simulink model "sampleModel267"  (R2021b)
settings: Solver=VariableStepAuto  StartTime=0.0  StopTime=10.0  RelTol=1e-3
undefined symbols (not defined in the file or in its folder): DiscIntNeverNeededParam, Newton, Raphson
libraries: simulink x5, slpidlib x1
settings Model: Creator=user  LastModifiedBy=user

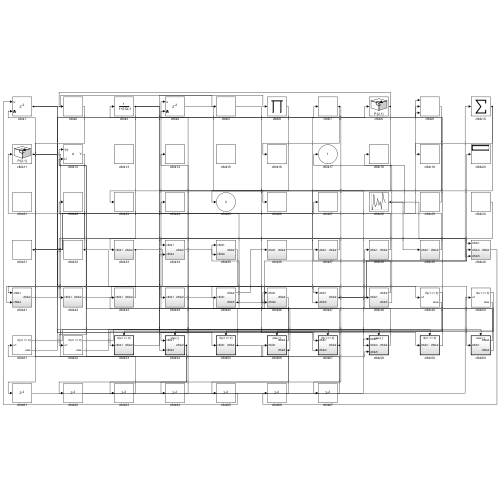
[thumbnail: Simulink's stored preview of the top-level diagram]
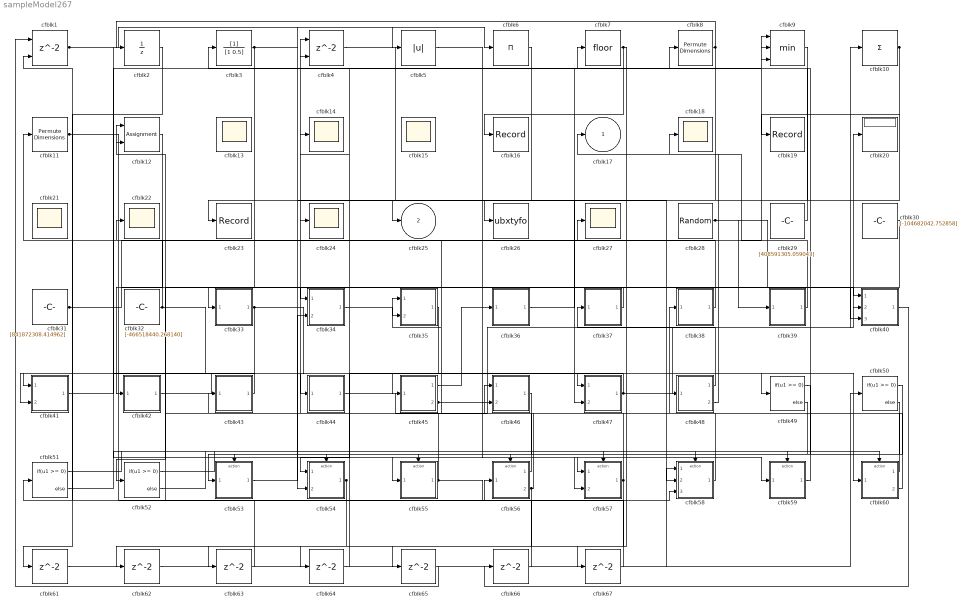
== system sampleModel267 ==
  cfblk1 : Delay  ShowEnablePort=on  SampleTime=1
      settings: InputPortMap=u0,e6
  cfblk10 : Sum  Inputs=+
  cfblk11 : PermuteDimensions
  cfblk12 : Assignment  DiagnosticForDimensions=Warning  IndexOptions=Index vector (dialog)  Indices=1  OutputSizes=1
  cfblk{13..15,18,21..22,24,27} (8 alike) : Scope
      cfblk13 settings: Floating=on
      cfblk15 settings: Floating=on
      cfblk21 settings: Floating=on
  cfblk16 : Record  FileSettingsInternal="{\"entries\":[{\"content\":{\"excelSettings\":{\"content\":{},\"type\":\"Streamout.ExcelSettings\"}},\"type\":\"Streamout.FileSettingStorage\",\"uuid\":\"38ef153d-d6ae-45e7-82f1-1ca2e326c5eb\"}],\"packageUris\":[\"http://schema.mathworks.com/mf0/streamout_blocks/R2020a\"],\"version\":\"1.0\"}"  SignalsInternal="{\"entries\":[{\"content\":{\"signals\":[{\"content\":{\"blockPath\":[\"sampleModel267/cfblk16\"],\"channel\":[],\"dimensions\":[1],\"domain\":\"sampleModel267/cfblk16\",\"lineColor\":\"#d95319\",\"plots\":[1],\"port\":1,\"sid\":[\"\"],\"signalID\":11134,\"signalName\":\"cfblk7\"},\"type\":\"RecordBlkView.Signal\",\"uuid\":\"f5056942-7931-4c3f-87a4-53e35f3bb4b1\"}]},\"type\":\"RecordBlkView.InputSignals\",\"uuid\":\"7db35bab-36c3-4b73-9a92-ac3f675e200d\"}],\"packageUris\":[\"http://schema.mathworks.com/mf0/streamout_blocks/R2020a\"],\"version\":\"1.0\"}"  VisualizationBindings="{\"sparklinesplugin\":{\"info\":[{\"bindingParametersList\":[],\"subplotID\":1}]}}"
  cfblk19 : Record  FileSettingsInternal="{\"entries\":[{\"content\":{\"excelSettings\":{\"content\":{},\"type\":\"Streamout.ExcelSettings\"}},\"type\":\"Streamout.FileSettingStorage\",\"uuid\":\"e67b9910-70a3-4f08-b618-b13b58853db8\"}],\"packageUris\":[\"http://schema.mathworks.com/mf0/streamout_blocks/R2020a\"],\"version\":\"1.0\"}"  SignalsInternal="{\"entries\":[{\"content\":{\"signals\":[{\"content\":{\"blockPath\":[\"sampleModel267/cfblk19\"],\"channel\":[],\"dimensions\":[1],\"domain\":\"sampleModel267/cfblk19\",\"lineColor\":\"#edb120\",\"plots\":[1],\"port\":1,\"sid\":[\"\"],\"signalID\":11138,\"signalName\":\"cfblk10\"},\"type\":\"RecordBlkView.Signal\",\"uuid\":\"ad1882d4-40aa-4b95-a06e-3b82c8a17900\"}]},\"type\":\"RecordBlkView.InputSignals\",\"uuid\":\"f4741eb0-9131-4b04-bfe2-4320a4acd3c2\"}],\"packageUris\":[\"http://schema.mathworks.com/mf0/streamout_blocks/R2020a\"],\"version\":\"1.0\"}"  VisualizationBindings="{\"sparklinesplugin\":{\"info\":[{\"bindingParametersList\":[],\"subplotID\":1}]}}"
  cfblk2 : UnitDelay  HasFrameUpgradeWarning=on
  cfblk20 : Display
  cfblk23 : Record  FileSettingsInternal="{\"entries\":[{\"content\":{\"excelSettings\":{\"content\":{},\"type\":\"Streamout.ExcelSettings\"}},\"type\":\"Streamout.FileSettingStorage\",\"uuid\":\"5cac87e1-3c50-4b70-acf6-de645cdb8377\"}],\"packageUris\":[\"http://schema.mathworks.com/mf0/streamout_blocks/R2020a\"],\"version\":\"1.0\"}"  SignalsInternal="{\"entries\":[{\"content\":{\"signals\":[{\"content\":{\"blockPath\":[\"sampleModel267/cfblk23\"],\"channel\":[],\"dimensions\":[1],\"domain\":\"sampleModel267/cfblk23\",\"lineColor\":\"#7e2f8e\",\"plots\":[1],\"port\":1,\"sid\":[\"\"],\"signalID\":11142,\"signalName\":\"cfblk10\"},\"type\":\"RecordBlkView.Signal\",\"uuid\":\"43345d3a-b4ac-4ed1-88fb-152ae4781999\"}]},\"type\":\"RecordBlkView.InputSignals\",\"uuid\":\"60e12632-78ef-4a34-abc7-bf1c9a5d24da\"}],\"packageUris\":[\"http://schema.mathworks.com/mf0/streamout_blocks/R2020a\"],\"version\":\"1.0\"}"  VisualizationBindings="{\"sparklinesplugin\":{\"info\":[{\"bindingParametersList\":[],\"subplotID\":1}]}}"
  cfblk26 : ToWorkspace  VariableName=ubxtyfo  SaveFormat=Timeseries  SampleTime=-1
  cfblk28 : UniformRandomNumber  Minimum=[-3933460180.447495]  Maximum=[5455943711.863254]  Seed=[92993268.000000]  SampleTime=0.1
  cfblk29 : Constant  Value=[408591305.059043]  SampleTime=1
  cfblk3 : DiscreteFilter  SampleTime=1
  cfblk30 : Constant  Value=[-104682042.752858]  SampleTime=1
  cfblk31 : Constant  Value=[841872308.414962]  SampleTime=1
  cfblk32 : Constant  Value=[-466518440.268140]  SampleTime=1
  cfblk33 : Subsystem
  cfblk34 : Subsystem
  cfblk35 : Subsystem
  cfblk36 : Subsystem
  cfblk37 : Subsystem
  cfblk38 : Subsystem
  cfblk39 : Subsystem
  cfblk4 : Delay  ShowEnablePort=on  SampleTime=1
      settings: InputPortMap=u0,e6
  cfblk40 : Subsystem
  cfblk41 : Subsystem
  cfblk42 : Subsystem
  cfblk43 : Subsystem
  cfblk44 : Subsystem
  cfblk45 : Subsystem
  cfblk46 : Subsystem
  cfblk47 : Subsystem
  cfblk48 : Subsystem
  cfblk{49..52} (4 alike) : If  IfExpression=u1 >= 0  SampleTime=1
  cfblk5 : Abs
  cfblk53 : Subsystem  TreatAsAtomicUnit=on
  cfblk54 : Subsystem  TreatAsAtomicUnit=on
  cfblk55 : Subsystem  TreatAsAtomicUnit=on
  cfblk56 : Subsystem  TreatAsAtomicUnit=on
  cfblk57 : Subsystem  TreatAsAtomicUnit=on
  cfblk58 : Subsystem  TreatAsAtomicUnit=on
  cfblk59 : Subsystem  TreatAsAtomicUnit=on
  cfblk6 : Product  Inputs=*
  cfblk60 : Subsystem  TreatAsAtomicUnit=on
  cfblk{61..67} (7 alike) : Delay  SampleTime=1
  cfblk7 : Rounding
  cfblk8 : PermuteDimensions
  cfblk9 : MinMax  Inputs=3
  cfblk17 : Outport
  cfblk25 : Outport  Port=2
  wires:
  cfblk7/1 -> cfblk16/1, cfblk67/1
  cfblk1/1 -> cfblk6/1, cfblk55/1(cfblk1), cfblk46/2(cfblk4)
  cfblk28/1 -> cfblk39/1(cfblk1), cfblk40/3(cfblk5)
  cfblk54/1(cfblk2) -> cfblk62/1, cfblk63/1
  cfblk11/1 -> cfblk56/1(cfblk1), cfblk57/1(cfblk1), cfblk9/3
  cfblk45/1(cfblk2) -> cfblk36/1(cfblk1)
  cfblk39/1(cfblk2) -> cfblk17/1
  cfblk46/1(cfblk2) -> cfblk53/1(cfblk1)
  cfblk44/1(cfblk2) -> cfblk60/1(cfblk1)
  cfblk5/1 -> cfblk59/1(cfblk1)
  cfblk59/1(cfblk2) -> cfblk9/1
  cfblk12/1 -> cfblk42/1(cfblk1)
  cfblk6/1 -> cfblk25/1
  cfblk29/1 -> cfblk3/1
  cfblk37/1(cfblk2) -> cfblk33/1(cfblk1)
  cfblk55/1(cfblk2) -> cfblk4/1, cfblk58/3(cfblk5)
  cfblk10/1 -> cfblk23/1, cfblk19/1
  cfblk60/1(cfblk2) -> cfblk38/1(cfblk1)
  cfblk8/1 -> cfblk2/1, cfblk54/2(cfblk3)
  cfblk30/1 -> cfblk34/1(cfblk1)
  cfblk48/1(cfblk2) -> cfblk37/1(cfblk1)
  cfblk47/1(cfblk2) -> cfblk45/1(cfblk1), cfblk10/1, cfblk40/2(cfblk4), cfblk48/1(cfblk1)
  cfblk36/1(cfblk2) -> cfblk8/1
  cfblk33/1(cfblk2) -> cfblk49/1, cfblk41/2(cfblk4)
  cfblk3/1 -> cfblk52/1, cfblk26/1, cfblk57/2(cfblk4), cfblk5/1
  cfblk42/1(cfblk2) -> cfblk47/1(cfblk1)
  cfblk56/1(cfblk2) -> cfblk35/1(cfblk1)
  cfblk32/1 -> cfblk44/1(cfblk1), cfblk22/1
  cfblk45/2(cfblk5) -> cfblk24/1, cfblk20/1
  cfblk43/1(cfblk2) -> cfblk41/1(cfblk1)
  cfblk56/2(cfblk5) -> cfblk46/1(cfblk1), cfblk64/1
  cfblk53/1(cfblk2) -> cfblk34/2(cfblk4)
  cfblk31/1 -> cfblk27/1, cfblk40/1(cfblk1), cfblk9/2
  cfblk4/1 -> cfblk58/2(cfblk4)
  cfblk48/2(cfblk3) -> cfblk18/1
  cfblk38/1(cfblk2) -> cfblk11/1
  cfblk60/2(cfblk4) -> cfblk43/1(cfblk1)
  cfblk58/1(cfblk2) -> cfblk12/1
  cfblk34/1(cfblk2) -> cfblk35/2(cfblk4)
  cfblk35/1(cfblk2) -> cfblk54/1(cfblk1)
  cfblk41/1(cfblk2) -> cfblk7/1
  cfblk57/1(cfblk2) -> cfblk14/1, cfblk65/1
  cfblk9/1 -> cfblk47/2(cfblk5)
  cfblk49/1 -> cfblk53/Action
  cfblk49/2 -> cfblk54/Action
  cfblk50/1 -> cfblk55/Action
  cfblk50/2 -> cfblk56/Action
  cfblk51/1 -> cfblk57/Action
  cfblk51/2 -> cfblk58/Action
  cfblk52/1 -> cfblk59/Action
  cfblk52/2 -> cfblk60/Action
  cfblk2/1 -> cfblk61/1
  cfblk61/1 -> cfblk50/1
  cfblk62/1 -> cfblk58/1(cfblk1)
  cfblk63/1 -> cfblk1/2
  cfblk64/1 -> cfblk4/2
  cfblk65/1 -> cfblk1/1
  cfblk40/1(cfblk2) -> cfblk66/1
  cfblk66/1 -> cfblk51/1
  cfblk67/1 -> cfblk12/2

== system sampleModel267/cfblk33 ==
  cfblk1 : Inport
  cfblk3 : simulink/Discrete/Tapped Delay  vinit=0.0  samptime=-1  NumDelays=1  DelayOrder=Oldest  includeCurrent=off
  cfblk4 : Sin  TimeSource=Use external signal  SampleTime=0
  cfblk2 : Outport
  wires:
  cfblk3/1 -> cfblk2/1
  cfblk1/1 -> cfblk4/1
  cfblk4/1 -> cfblk3/1

== system sampleModel267/cfblk34 ==
  cfblk1 : Inport
  cfblk4 : Inport  Port=2
  cfblk3 : Product  Inputs=*
  cfblk2 : Outport
  wires:
  cfblk4/1 -> cfblk3/1
  cfblk3/1 -> cfblk2/1

== system sampleModel267/cfblk35 ==
  cfblk1 : Inport
  cfblk4 : Inport  Port=2
  cfblk3 : MinMax  Function=max  Inputs=3
  cfblk2 : Outport
  wires:
  cfblk4/1 -> cfblk2/1, cfblk3/2
  cfblk1/1 -> cfblk3/1, cfblk3/3

== system sampleModel267/cfblk36 ==
  cfblk1 : Inport
  cfblk3 : UnaryMinus
  cfblk4 : PermuteDimensions
  cfblk2 : Outport
  wires:
  cfblk3/1 -> cfblk4/1
  cfblk4/1 -> cfblk2/1
  cfblk1/1 -> cfblk3/1

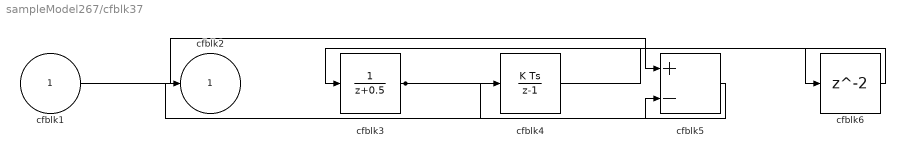
== system sampleModel267/cfblk37 ==
  cfblk1 : Inport
  cfblk3 : DiscreteTransferFcn  SampleTime=1
  cfblk4 : DiscreteIntegrator  ICPrevOutput=DiscIntNeverNeededParam  ICPrevScaledInput=DiscIntNeverNeededParam
  cfblk5 : Sum  Inputs=+-
  cfblk6 : Delay  SampleTime=1
  cfblk2 : Outport
  wires:
  cfblk3/1 -> cfblk4/1, cfblk5/2
  cfblk1/1 -> cfblk5/1
  cfblk5/1 -> cfblk2/1
  cfblk4/1 -> cfblk6/1
  cfblk6/1 -> cfblk3/1

== system sampleModel267/cfblk38 ==
  cfblk1 : Inport
  cfblk3 : simulink/Math Operations/MinMax Running Resettable  Function=min  vinit=0.0
  cfblk4 : Constant  Value=[-534675047.013126]  SampleTime=1
  cfblk2 : Outport
  wires:
  cfblk1/1 -> cfblk3/1
  cfblk4/1 -> cfblk3/2
  cfblk3/1 -> cfblk2/1

== system sampleModel267/cfblk39 ==
  cfblk1 : Inport
  cfblk3 : Bias  Bias=[-354064516.958488]
  cfblk2 : Outport
  wires:
  cfblk1/1 -> cfblk3/1
  cfblk3/1 -> cfblk2/1

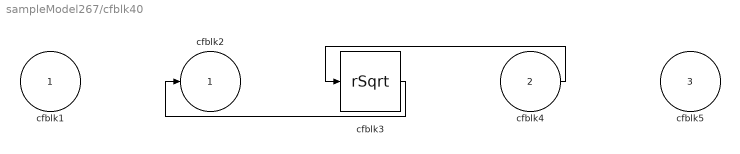
== system sampleModel267/cfblk40 ==
  cfblk1 : Inport
  cfblk4 : Inport  Port=2
  cfblk5 : Inport  Port=3
  cfblk3 : Sqrt  Operator=rSqrt  AlgorithmType=Newton-Raphson  SaturateOnIntegerOverflow=on
  cfblk2 : Outport
  wires:
  cfblk4/1 -> cfblk3/1
  cfblk3/1 -> cfblk2/1

== system sampleModel267/cfblk41 ==
  cfblk1 : Inport
  cfblk4 : Inport  Port=2
  cfblk3 : simulink/Discrete/Difference  ICPrevInput=0.0  OutMin=[]  OutMax=[]  OutDataTypeStr=Inherit: Inherit via back propagation  OutDataType=fixdt(1, 16)  OutScaling=2^-10  DoSatur=off
  cfblk2 : Outport
  wires:
  cfblk4/1 -> cfblk3/1
  cfblk1/1 -> cfblk2/1

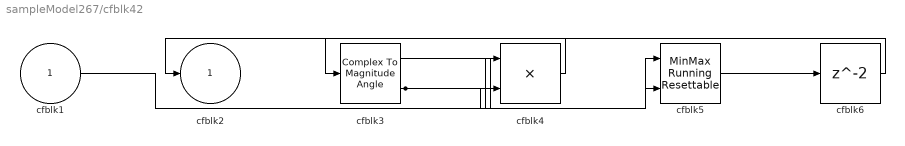
== system sampleModel267/cfblk42 ==
  cfblk1 : Inport
  cfblk3 : ComplexToMagnitudeAngle
  cfblk4 : Product  Inputs=**
  cfblk5 : simulink/Math Operations/MinMax Running Resettable  Function=min  vinit=0.0
  cfblk6 : Delay  SampleTime=1
  cfblk2 : Outport
  wires:
  cfblk4/1 -> cfblk2/1
  cfblk3/1 -> cfblk5/1
  cfblk1/1 -> cfblk4/1
  cfblk3/2 -> cfblk4/2, cfblk5/2
  cfblk5/1 -> cfblk6/1
  cfblk6/1 -> cfblk3/1

== system sampleModel267/cfblk43 ==
  cfblk1 : Inport
  cfblk3 : simulink/Discrete/Transfer Fcn First Order  PoleZ=0.95  ICPrevOutput=0.0  DoSatur=off
  cfblk2 : Outport
  wires:
  cfblk1/1 -> cfblk3/1
  cfblk3/1 -> cfblk2/1

== system sampleModel267/cfblk44 ==
  cfblk1 : Inport
  cfblk3 : DiscreteFilter  SampleTime=1
  cfblk4 : Product
  cfblk2 : Outport
  wires:
  cfblk3/1 -> cfblk2/1, cfblk4/1
  cfblk1/1 -> cfblk3/1, cfblk4/2

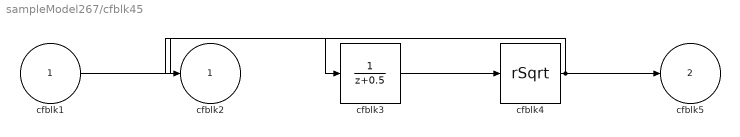
== system sampleModel267/cfblk45 ==
  cfblk1 : Inport
  cfblk3 : DiscreteTransferFcn  SampleTime=1
  cfblk4 : Sqrt  Operator=rSqrt  AlgorithmType=Newton-Raphson  SaturateOnIntegerOverflow=on
  cfblk2 : Outport
  cfblk5 : Outport  Port=2
  wires:
  cfblk1/1 -> cfblk3/1
  cfblk3/1 -> cfblk4/1
  cfblk4/1 -> cfblk5/1, cfblk2/1

== system sampleModel267/cfblk46 ==
  cfblk1 : Inport
  cfblk4 : Inport  Port=2
  cfblk3 : ComplexToMagnitudeAngle
  cfblk2 : Outport
  wires:
  cfblk4/1 -> cfblk3/1
  cfblk3/1 -> cfblk2/1

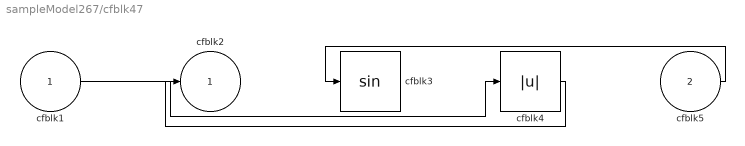
== system sampleModel267/cfblk47 ==
  cfblk1 : Inport
  cfblk5 : Inport  Port=2
  cfblk3 : Trigonometry
  cfblk4 : Abs
  cfblk2 : Outport
  wires:
  cfblk5/1 -> cfblk3/1
  cfblk1/1 -> cfblk4/1
  cfblk4/1 -> cfblk2/1

== system sampleModel267/cfblk48 ==
  cfblk1 : Inport
  cfblk2 : Outport
  cfblk3 : Outport  Port=2
  wires:
  cfblk1/1 -> cfblk2/1, cfblk3/1

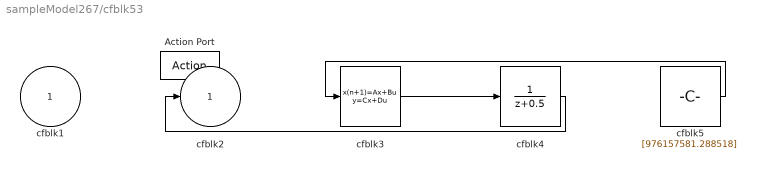
== system sampleModel267/cfblk53 ==
  cfblk1 : Inport
  Action Port : ActionPort  ActionPortLabel=if(u1 >= 0)
  cfblk3 : DiscreteStateSpace  SampleTime=-1
  cfblk4 : DiscreteTransferFcn
  cfblk5 : Constant  Value=[976157581.288518]  SampleTime=1
  cfblk2 : Outport
  wires:
  cfblk4/1 -> cfblk2/1
  cfblk5/1 -> cfblk3/1
  cfblk3/1 -> cfblk4/1

== system sampleModel267/cfblk54 ==
  cfblk1 : Inport
  cfblk3 : Inport  Port=2
  Action Port : ActionPort  ActionPortLabel=else
  cfblk2 : Outport
  wires:
  cfblk3/1 -> cfblk2/1

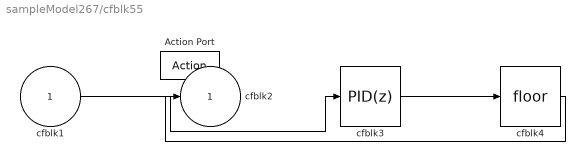
== system sampleModel267/cfblk55 ==
  cfblk1 : Inport
  Action Port : ActionPort  ActionPortLabel=if(u1 >= 0)
  cfblk3 : slpidlib/PID Controller  Controller=PID  Form=Parallel  TimeDomain=Discrete-time  UseExternalTs=off  SampleTime=-1  IntegratorMethod=Forward Euler  FilterMethod=Forward Euler  ControllerParametersSource=internal  P=1  I=1  D=0  UseFilter=on  N=100  TunerSelectOption=Transfer Function Based (PID Tuner App)  InitialConditionSource=internal  InitialConditionForIntegrator=0  InitialConditionForFilter=0  DifferentiatorICPrevScaledInput=0  ExternalReset=none  TrackingMode=off  Kt=1  LimitOutput=off  SatLimitsSource=internal  UpperSaturationLimit=inf  LowerSaturationLimit=-inf  LinearizeAsGain=off  AntiWindupMode=none  Kb=1  POutMin=[]  POutMax=[]  IOutMin=[]  IOutMax=[]  DOutMin=[]  DOutMax=[]  NOutMin=[]  NOutMax=[]  SumOutMin=[]  SumOutMax=[]  SaturationOutMin=[]  SaturationOutMax=[]  PParamMin=[]  PParamMax=[]  IParamMin=[]  IParamMax=[]  DParamMin=[]  DParamMax=[]  NParamMin=[]  NParamMax=[]  KbParamMin=[]  KbParamMax=[]  KtParamMin=[]  KtParamMax=[]  KbOutMin=[]  KbOutMax=[]  KtOutMin=[]  KtOutMax=[]  IntegratorOutMin=[]  IntegratorOutMax=[]  FilterOutMin=[]  FilterOutMax=[]  SumI1OutMin=[]  SumI1OutMax=[]  SumI2OutMin=[]  SumI2OutMax=[]  SumI3OutMin=[]  SumI3OutMax=[]  SumI4OutMin=[]  SumI4OutMax=[]  SumDOutMin=[]  SumDOutMax=[]  DifferentiatorOutMin=[]  DifferentiatorOutMax=[]  FilterDiffOutCoefMin=[]  FilterDiffOutCoefMax=[]  ReciprocalOutMin=[]  ReciprocalOutMax=[]  SumDenOutMin=[]  SumDenOutMax=[]  SumNumOutMin=[]  SumNumOutMax=[]  DivideOutMin=[]  DivideOutMax=[]  UdiffTsProdOutMin=[]  UdiffTsProdOutMax=[]  NTsProdOutMin=[]  NTsProdOutMax=[]  UintegralTsProdOutMin=[]  UintegralTsProdOutMax=[]  UngainTsProdOutMin=[]  UngainTsProdOutMax=[]  IntegratorContinuousStateAttributes=''  IntegratorStateMustResolveToSignalObject=off  IntegratorRTWStateStorageClass=Auto  FilterContinuousStateAttributes=''  FilterStateMustResolveToSignalObject=off  FilterRTWStateStorageClass=Auto  ParallelPVariant=InternalParameters  IdealPVariant=Disabled  IVariant=InternalParameters  DVariant=InternalParameters  IntegratorVariant=Discrete  SatVariant=Disabled  AWVariant=Passthrough  PCopyVariant=Disabled  TRVariant=Disabled  FdbkBlocksVariant=Forward  IdealPFdbkVariant=Disabled  SatFdbkVariant=Disabled  DerivativeFilterVariant=ForwardEulerFilter  NVariant=InternalParameters  NCopyVariant=Disabled  FilterICVariant=InternalICsFilter  IntegratorICVariant=InternalICs  ExternalResetVariant=Disabled  TRSumVariant=Passthrough  SumFdbkVariant=Disabled  SumVariant=Sum_PID  TsampFilterVariant=InternalTs  TsampNgainVariant=Passthrough  TsampIntegralVariant=Passthrough  ExternalSaturationOutDataTypeStr=Inherit: Same as second input
  cfblk4 : Rounding
  cfblk2 : Outport
  wires:
  cfblk1/1 -> cfblk3/1
  cfblk3/1 -> cfblk4/1
  cfblk4/1 -> cfblk2/1

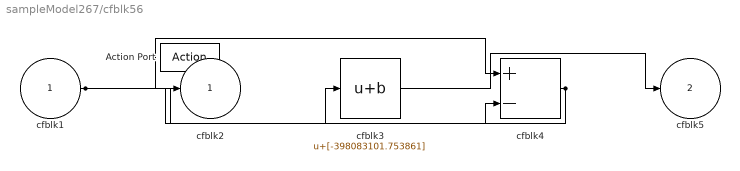
== system sampleModel267/cfblk56 ==
  cfblk1 : Inport
  Action Port : ActionPort  ActionPortLabel=else
  cfblk3 : Bias  Bias=[-398083101.753861]
  cfblk4 : Sum  Inputs=+-
  cfblk2 : Outport
  cfblk5 : Outport  Port=2
  wires:
  cfblk3/1 -> cfblk5/1
  cfblk1/1 -> cfblk4/1, cfblk4/2
  cfblk4/1 -> cfblk3/1, cfblk2/1

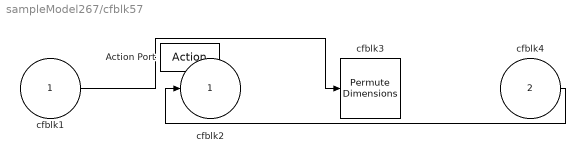
== system sampleModel267/cfblk57 ==
  cfblk1 : Inport
  cfblk4 : Inport  Port=2
  Action Port : ActionPort  ActionPortLabel=if(u1 >= 0)
  cfblk3 : PermuteDimensions
  cfblk2 : Outport
  wires:
  cfblk4/1 -> cfblk2/1
  cfblk1/1 -> cfblk3/1

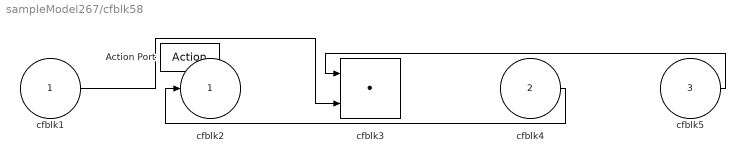
== system sampleModel267/cfblk58 ==
  cfblk1 : Inport
  cfblk4 : Inport  Port=2
  cfblk5 : Inport  Port=3
  Action Port : ActionPort  ActionPortLabel=else
  cfblk3 : DotProduct  InputSameDT=on  OutDataTypeStr=Inherit: Inherit via internal rule
  cfblk2 : Outport
  wires:
  cfblk4/1 -> cfblk2/1
  cfblk5/1 -> cfblk3/1
  cfblk1/1 -> cfblk3/2

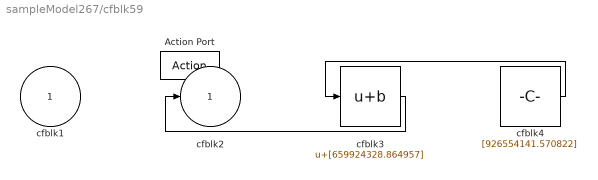
== system sampleModel267/cfblk59 ==
  cfblk1 : Inport
  Action Port : ActionPort  ActionPortLabel=if(u1 >= 0)
  cfblk3 : Bias  Bias=[659924328.864957]
  cfblk4 : Constant  Value=[926554141.570822]  SampleTime=1
  cfblk2 : Outport
  wires:
  cfblk3/1 -> cfblk2/1
  cfblk4/1 -> cfblk3/1

== system sampleModel267/cfblk60 ==
  cfblk1 : Inport
  Action Port : ActionPort  ActionPortLabel=else
  cfblk3 : Product  Inputs=*
  cfblk2 : Outport
  cfblk4 : Outport  Port=2
  wires:
  cfblk1/1 -> cfblk3/1, cfblk4/1
  cfblk3/1 -> cfblk2/1
